simulink model "Control_cascada_PID_feedfoward_antiwindup_smith"  (R2019a)
settings: Solver=VariableStepAuto  StartTime=0.0  StopTime=600  RelTol=1e-3
libraries: simulink x6
settings Model: Creator=Alejoxbg  LastModifiedBy=Alejoxbg

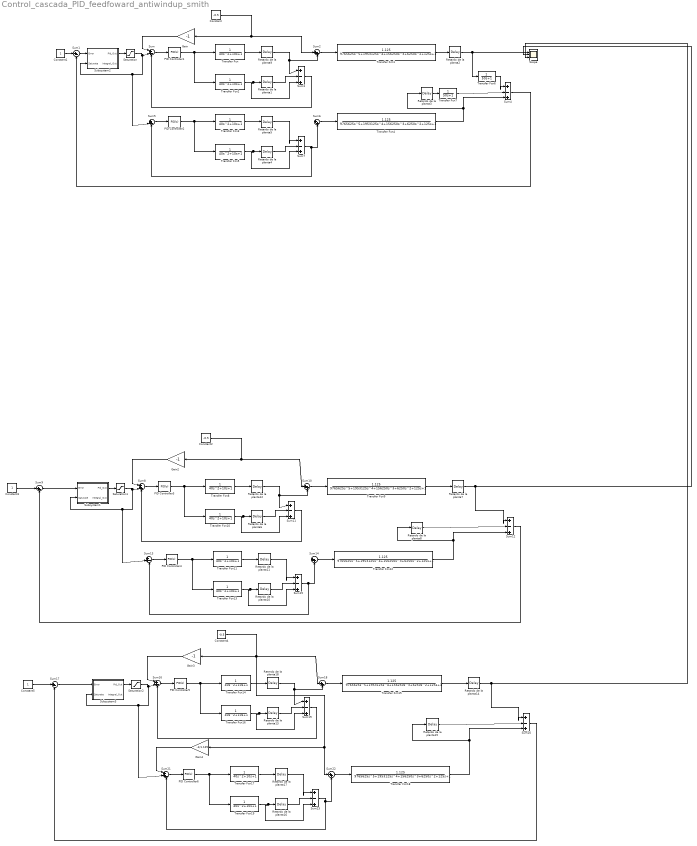
== system Control_cascada_PID_feedfoward_antiwindup_smith ==
  Constant : Constant  Value=-0.5
  Constant1 : Constant
  Constant2 : Constant  Value=-0.5
  Constant3 : Constant
  Constant4 : Constant  Value=-0.5
  Constant5 : Constant
  Gain : Gain  Gain=-1
  Gain2 : Gain  Gain=-1
  Gain3 : Gain  Gain=-1
  Gain4 : Gain  Gain=-1/1.125
  PID Controller{1..6} (6 alike) : simulink/Continuous/PID Controller  Controller=PID  Form=Parallel  TimeDomain=Continuous-time  SampleTime=-1  IntegratorMethod=Forward Euler  FilterMethod=Forward Euler  ControllerParametersSource=internal  P=12.1148539818802  I=1.25631014904339  D=27.6845650272969  UseFilter=on  N=4.3146205312046  TunerSelectOption=Transfer Function Based (PID Tuner App)  InitialConditionSource=internal  InitialConditionForIntegrator=0  InitialConditionForFilter=0  DifferentiatorICPrevScaledInput=0  ExternalReset=none  TrackingMode=off  Kt=1  LimitOutput=off  UpperSaturationLimit=inf  LowerSaturationLimit=-inf  LinearizeAsGain=on  AntiWindupMode=none  Kb=1  POutMin=[]  POutMax=[]  IOutMin=[]  IOutMax=[]  DOutMin=[]  DOutMax=[]  NOutMin=[]  NOutMax=[]  SumOutMin=[]  SumOutMax=[]  SaturationOutMin=[]  SaturationOutMax=[]  PParamMin=[]  PParamMax=[]  IParamMin=[]  IParamMax=[]  DParamMin=[]  DParamMax=[]  NParamMin=[]  NParamMax=[]  KbParamMin=[]  KbParamMax=[]  KtParamMin=[]  KtParamMax=[]  KbOutMin=[]  KbOutMax=[]  KtOutMin=[]  KtOutMax=[]  IntegratorOutMin=[]  IntegratorOutMax=[]  FilterOutMin=[]  FilterOutMax=[]  SumI1OutMin=[]  SumI1OutMax=[]  SumI2OutMin=[]  SumI2OutMax=[]  SumI3OutMin=[]  SumI3OutMax=[]  SumI4OutMin=[]  SumI4OutMax=[]  SumDOutMin=[]  SumDOutMax=[]  DifferentiatorOutMin=[]  DifferentiatorOutMax=[]  FilterDiffOutCoefMin=[]  FilterDiffOutCoefMax=[]  ReciprocalOutMin=[]  ReciprocalOutMax=[]  SumDenOutMin=[]  SumDenOutMax=[]  SumNumOutMin=[]  SumNumOutMax=[]  DivideOutMin=[]  DivideOutMax=[]  IntegratorContinuousStateAttributes=''  IntegratorStateMustResolveToSignalObject=off  IntegratorRTWStateStorageClass=Auto  FilterContinuousStateAttributes=''  FilterStateMustResolveToSignalObject=off  FilterRTWStateStorageClass=Auto  ParallelPVariant=InternalParameters  IdealPVariant=Disabled  IVariant=InternalParameters  DVariant=InternalParameters  IntegratorVariant=Continuous  SatVariant=Disabled  AWVariant=Passthrough  PCopyVariant=Disabled  TRVariant=Disabled  FdbkBlocksVariant=Forward  IdealPFdbkVariant=Disabled  SatFdbkVariant=Disabled  DerivativeFilterVariant=ContFilter  NVariant=InternalParameters  NCopyVariant=Disabled  FilterICVariant=InternalICsFilter  IntegratorICVariant=InternalICs  ExternalResetVariant=Disabled  TRSumVariant=Passthrough  SumFdbkVariant=Disabled  SumVariant=Sum_PID
  Retardo de la planta{1..18} (18 alike) : TransportDelay  DelayTime=10
  Saturation : Saturate  UpperLimit=1  LowerLimit=-1  ZeroCross=off
  Saturation1 : Saturate  UpperLimit=1  LowerLimit=-1  ZeroCross=off
  Saturation2 : Saturate  UpperLimit=1  LowerLimit=-1  ZeroCross=off
  Scope : Scope  NumInputPorts=3
  Subsystem1 : Subsystem  mask{Kp=1.04993394811551, Ki=0.0105409170991703, Kd=19.9679501950648, Kt=10}
      mask help: PID with anti wind up
  Subsystem2 : Subsystem  mask{Kp=1.04993394811551, Ki=0.0105409170991703, Kd=19.9679501950648, Kt=10}
      mask help: PID with anti wind up
  Subsystem3 : Subsystem  mask{Kp=1.04993394811551, Ki=0.0105409170991703, Kd=19.9679501950648, Kt=10}
      mask help: PID with anti wind up
  Sum{,5,8,13,16,21} (6 alike) : Sum  Inputs=|++-
  Sum1 : Sum  Inputs=|+-
  Sum{2,6,10,14,18,22} (6 alike) : Sum  Inputs=|++
  Sum{3..4,7,11..12,15,19..20,23} (9 alike) : Sum  Inputs=|+-+
  Sum17 : Sum  Inputs=|+-
  Sum9 : Sum  Inputs=|+-
  Transfer Fcn{,2..3,5,8,10..11,13..14,16..17,19} (12 alike) : TransferFcn  Denominator=[40 10 1]
  Transfer Fcn{1,4,9,12,15,18} (6 alike) : TransferFcn  Numerator=[1.125]  Denominator="[9765625     1953125      156250        6250         125           1 ]"
  Transfer Fcn6 : TransferFcn  Denominator=[50,1]
  Transfer Fcn7 : TransferFcn  Denominator=[50,1]
  wires:
  Constant1/1 -> Sum1/1
  Sum1/1 -> Subsystem2/1(Error)
  Gain/1 -> Sum/1
  Sum/1 -> PID Controller1/1
  Sum2/1 -> Transfer Fcn1/1
  PID Controller1/1 -> Transfer Fcn2/1, Transfer Fcn/1
  Subsystem2/1(Pid_Out) -> Saturation/1
  Transfer Fcn/1 -> Retardo de la planta9/1
  Transfer Fcn2/1 -> Sum3/3, Retardo de la planta1/1
  Retardo de la planta9/1 -> Sum2/2, Sum3/1
  Retardo de la planta1/1 -> Sum3/2
  Sum3/1 -> Sum/3
  Retardo de la planta2/1 -> Scope/1, Transfer Fcn6/1
  Transfer Fcn1/1 -> Retardo de la planta2/1
  Sum4/1 -> Sum1/2
  Retardo de la planta4/1 -> Sum7/2
  Sum7/1 -> Sum6/2, Sum5/3
  Constant/1 -> Sum2/1, Gain/1
  Retardo de la planta5/1 -> Sum7/1
  Transfer Fcn5/1 -> Sum7/3, Retardo de la planta4/1
  Transfer Fcn3/1 -> Retardo de la planta5/1
  Sum6/1 -> Transfer Fcn4/1
  PID Controller2/1 -> Transfer Fcn5/1, Transfer Fcn3/1
  Saturation/1 -> Sum5/2, Subsystem2/2(Saturate), Sum/2
  Sum5/1 -> PID Controller2/1
  Transfer Fcn4/1 -> Retardo de la planta3/1, Sum4/3
  Transfer Fcn6/1 -> Sum4/1
  Transfer Fcn7/1 -> Sum4/2
  Retardo de la planta3/1 -> Transfer Fcn7/1
  Sum8/1 -> PID Controller3/1
  Sum15/1 -> Sum14/2, Sum13/3
  Sum9/1 -> Subsystem1/1(Error)
  Transfer Fcn8/1 -> Retardo de la planta12/1
  Sum14/1 -> Transfer Fcn12/1
  Sum10/1 -> Transfer Fcn9/1
  Transfer Fcn9/1 -> Retardo de la planta7/1
  Sum12/1 -> Sum9/2
  Retardo de la planta10/1 -> Sum15/2
  Transfer Fcn10/1 -> Sum11/3, Retardo de la planta6/1
  Transfer Fcn11/1 -> Retardo de la planta11/1
  Gain2/1 -> Sum8/1
  Transfer Fcn12/1 -> Sum12/3, Retardo de la planta8/1
  Subsystem1/1(Pid_Out) -> Saturation1/1
  Sum13/1 -> PID Controller4/1
  Constant3/1 -> Sum9/1
  Transfer Fcn13/1 -> Sum15/3, Retardo de la planta10/1
  Saturation1/1 -> Sum13/2, Subsystem1/2(Saturate), Sum8/2
  Retardo de la planta6/1 -> Sum11/2
  Retardo de la planta12/1 -> Sum10/2, Sum11/1
  Retardo de la planta11/1 -> Sum15/1
  PID Controller4/1 -> Transfer Fcn13/1, Transfer Fcn11/1
  Constant2/1 -> Sum10/1, Gain2/1
  Retardo de la planta7/1 -> Scope/2, Sum12/1
  PID Controller3/1 -> Transfer Fcn10/1, Transfer Fcn8/1
  Retardo de la planta8/1 -> Sum12/2
  Retardo de la planta14/1 -> Sum20/1, Scope/3
  Constant5/1 -> Sum17/1
  Retardo de la planta17/1 -> Sum23/1
  Sum20/1 -> Sum17/2
  Retardo de la planta15/1 -> Sum20/2
  PID Controller6/1 -> Transfer Fcn19/1, Transfer Fcn17/1
  Transfer Fcn17/1 -> Retardo de la planta17/1
  Sum16/1 -> PID Controller5/1
  Constant4/1 -> Gain4/1, Sum22/1, Sum18/1, Gain3/1
  Subsystem3/1(Pid_Out) -> Saturation2/1
  Transfer Fcn19/1 -> Sum23/3, Retardo de la planta16/1
  Retardo de la planta16/1 -> Sum23/2
  Retardo de la planta13/1 -> Sum19/2
  Saturation2/1 -> Sum21/2, Subsystem3/2(Saturate), Sum16/2
  Transfer Fcn16/1 -> Sum19/3, Retardo de la planta13/1
  Sum19/1 -> Sum16/3
  Gain3/1 -> Sum16/1
  Sum23/1 -> Sum22/2, Sum21/3
  Sum17/1 -> Subsystem3/1(Error)
  Sum22/1 -> Transfer Fcn18/1
  Sum18/1 -> Transfer Fcn15/1
  Transfer Fcn14/1 -> Retardo de la planta18/1
  Transfer Fcn18/1 -> Retardo de la planta15/1, Sum20/3
  PID Controller5/1 -> Transfer Fcn16/1, Transfer Fcn14/1
  Sum21/1 -> PID Controller6/1
  Gain4/1 -> Sum21/1
  Retardo de la planta18/1 -> Sum18/2, Sum19/1
  Transfer Fcn15/1 -> Retardo de la planta14/1
  Sum11/1 -> Sum8/3

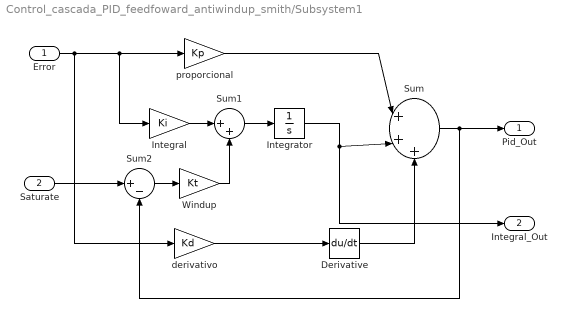
== system Control_cascada_PID_feedfoward_antiwindup_smith/Subsystem1 ==
  Error : Inport
  Saturate : Inport  Port=2
  Derivative : Derivative
  Integral : Gain  Gain=Ki  SaturateOnIntegerOverflow=on  OutDataTypeStr=Inherit: Same as input  ParamDataTypeStr=Inherit: Same as input
  Integrator : Integrator
  Sum : Sum  Inputs=|+++  SaturateOnIntegerOverflow=on  InputSameDT=on  OutDataTypeStr=Inherit: Same as first input
  Sum1 : Sum  Inputs=|++  SaturateOnIntegerOverflow=on  InputSameDT=on  OutDataTypeStr=Inherit: Same as first input
  Sum2 : Sum  Inputs=|+-  SaturateOnIntegerOverflow=on  InputSameDT=on  OutDataTypeStr=Inherit: Same as first input
  Windup : Gain  Gain=Kt  SaturateOnIntegerOverflow=on  OutDataTypeStr=Inherit: Same as input  ParamDataTypeStr=Inherit: Same as input
  derivativo : Gain  Gain=Kd  SaturateOnIntegerOverflow=on  OutDataTypeStr=Inherit: Same as input  ParamDataTypeStr=Inherit: Same as input
  proporcional : Gain  Gain=Kp  SaturateOnIntegerOverflow=on  OutDataTypeStr=Inherit: Same as input  ParamDataTypeStr=Inherit: Same as input
  Pid_Out : Outport
  Integral_Out : Outport  Port=2
  wires:
  Error/1 -> Integral/1, proporcional/1, derivativo/1
  Sum/1 -> Pid_Out/1, Sum2/2
  Integrator/1 -> Sum/2, Integral_Out/1
  proporcional/1 -> Sum/1
  Derivative/1 -> Sum/3
  Integral/1 -> Sum1/1
  Sum1/1 -> Integrator/1
  Windup/1 -> Sum1/2
  Saturate/1 -> Sum2/1
  Sum2/1 -> Windup/1
  derivativo/1 -> Derivative/1

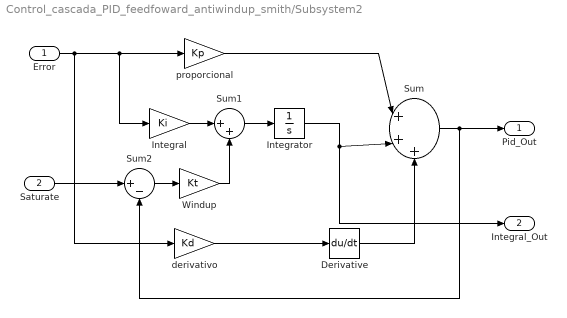
== system Control_cascada_PID_feedfoward_antiwindup_smith/Subsystem2 ==
  Error : Inport
  Saturate : Inport  Port=2
  Derivative : Derivative
  Integral : Gain  Gain=Ki  SaturateOnIntegerOverflow=on  OutDataTypeStr=Inherit: Same as input  ParamDataTypeStr=Inherit: Same as input
  Integrator : Integrator
  Sum : Sum  Inputs=|+++  SaturateOnIntegerOverflow=on  InputSameDT=on  OutDataTypeStr=Inherit: Same as first input
  Sum1 : Sum  Inputs=|++  SaturateOnIntegerOverflow=on  InputSameDT=on  OutDataTypeStr=Inherit: Same as first input
  Sum2 : Sum  Inputs=|+-  SaturateOnIntegerOverflow=on  InputSameDT=on  OutDataTypeStr=Inherit: Same as first input
  Windup : Gain  Gain=Kt  SaturateOnIntegerOverflow=on  OutDataTypeStr=Inherit: Same as input  ParamDataTypeStr=Inherit: Same as input
  derivativo : Gain  Gain=Kd  SaturateOnIntegerOverflow=on  OutDataTypeStr=Inherit: Same as input  ParamDataTypeStr=Inherit: Same as input
  proporcional : Gain  Gain=Kp  SaturateOnIntegerOverflow=on  OutDataTypeStr=Inherit: Same as input  ParamDataTypeStr=Inherit: Same as input
  Pid_Out : Outport
  Integral_Out : Outport  Port=2
  wires:
  Error/1 -> Integral/1, proporcional/1, derivativo/1
  Sum/1 -> Pid_Out/1, Sum2/2
  Integrator/1 -> Sum/2, Integral_Out/1
  proporcional/1 -> Sum/1
  Derivative/1 -> Sum/3
  Integral/1 -> Sum1/1
  Sum1/1 -> Integrator/1
  Windup/1 -> Sum1/2
  Saturate/1 -> Sum2/1
  Sum2/1 -> Windup/1
  derivativo/1 -> Derivative/1

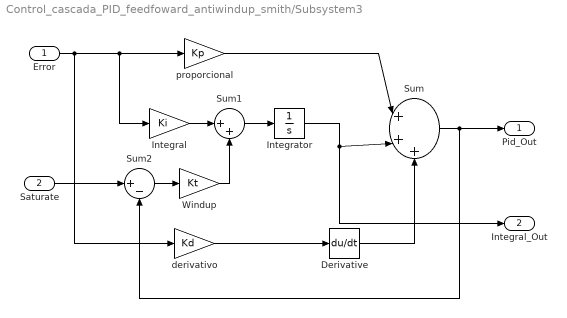
== system Control_cascada_PID_feedfoward_antiwindup_smith/Subsystem3 ==
  Error : Inport
  Saturate : Inport  Port=2
  Derivative : Derivative
  Integral : Gain  Gain=Ki  SaturateOnIntegerOverflow=on  OutDataTypeStr=Inherit: Same as input  ParamDataTypeStr=Inherit: Same as input
  Integrator : Integrator
  Sum : Sum  Inputs=|+++  SaturateOnIntegerOverflow=on  InputSameDT=on  OutDataTypeStr=Inherit: Same as first input
  Sum1 : Sum  Inputs=|++  SaturateOnIntegerOverflow=on  InputSameDT=on  OutDataTypeStr=Inherit: Same as first input
  Sum2 : Sum  Inputs=|+-  SaturateOnIntegerOverflow=on  InputSameDT=on  OutDataTypeStr=Inherit: Same as first input
  Windup : Gain  Gain=Kt  SaturateOnIntegerOverflow=on  OutDataTypeStr=Inherit: Same as input  ParamDataTypeStr=Inherit: Same as input
  derivativo : Gain  Gain=Kd  SaturateOnIntegerOverflow=on  OutDataTypeStr=Inherit: Same as input  ParamDataTypeStr=Inherit: Same as input
  proporcional : Gain  Gain=Kp  SaturateOnIntegerOverflow=on  OutDataTypeStr=Inherit: Same as input  ParamDataTypeStr=Inherit: Same as input
  Pid_Out : Outport
  Integral_Out : Outport  Port=2
  wires:
  Error/1 -> Integral/1, proporcional/1, derivativo/1
  Sum/1 -> Pid_Out/1, Sum2/2
  Integrator/1 -> Sum/2, Integral_Out/1
  proporcional/1 -> Sum/1
  Derivative/1 -> Sum/3
  Integral/1 -> Sum1/1
  Sum1/1 -> Integrator/1
  Windup/1 -> Sum1/2
  Saturate/1 -> Sum2/1
  Sum2/1 -> Windup/1
  derivativo/1 -> Derivative/1
